simulink model "c7mlor1b"  (Simulink 7.7)
settings: Solver=ode45  StartTime=0.0  StopTime=10.0  RelTol=1e-7
PreLoadFcn:
  | beta=8/3; rho=10; sigma=28;
settings Model: Creator=Professor Dingyu Xue  LastModifiedBy=Professor Dingyu Xue
settings DataIOCC: SignalLoggingName=sigsOut
settings DebuggingCC: SaveWithParameterizedLinksMsg=none  SignalResolutionControl=TryResolveAllWithWarning  SolverPrmCheckMsg=none  MultiTaskDSMMsg=warning  MultiTaskCondExecSysMsg=none  StrictBusMsg=None
settings HardwareCC: TargetUnknown=on
settings RTWCC: IncludeERTFirstTime=on

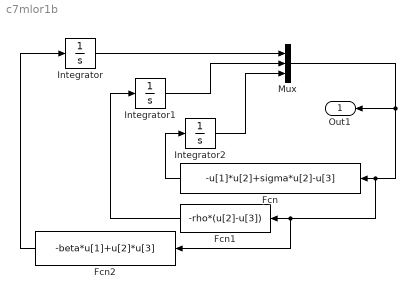
== system c7mlor1b ==
  Fcn : Fcn  Expr=-u[1]*u[2]+sigma*u[2]-u[3]
  Fcn1 : Fcn  Expr=-rho*(u[2]-u[3])
  Fcn2 : Fcn  Expr=-beta*u[1]+u[2]*u[3]
  Integrator : Integrator
  Integrator1 : Integrator
  Integrator2 : Integrator  InitialCondition=1e-3
  Mux : Mux  Inputs=3
  Out1 : Outport
  wires:
  Integrator/1 -> Mux/1
  Integrator1/1 -> Mux/2
  Integrator2/1 -> Mux/3
  Mux/1 -> Fcn/1, Fcn1/1, Fcn2/1, Out1/1
  Fcn/1 -> Integrator2/1
  Fcn1/1 -> Integrator1/1
  Fcn2/1 -> Integrator/1
